simulink model "pi_seqOfFixedSizeIface"  (R2018b)
settings: Solver=FixedStepDiscrete  StartTime=0.0  StopTime=10.0  RelTol=1e-3
settings Model: Creator=matlab  LastModifiedBy=matlab
settings DataIOCC: SaveOutput=off  SignalLogging=off  SaveTime=off
settings OptimizationCC: DefaultParameterBehavior=Inlined  EnhancedBackFolding=on  PassReuseOutputArgsAs=Individual arguments  OptimizeBlockOrder=speed  DifferentSizesBufferReuse=on  OptimizationCustomize=off
settings DebuggingCC: ParameterTunabilityLossMsg=error
settings SFSimCC: MATLABDynamicMemAlloc=off
settings RTWCC: SystemTargetFile=ert.tlc  TemplateMakefile=ert_default_tmf  PostCodeGenCommand=packNGo(buildInfo);  GenerateReport=on  IncludeHyperlinkInReport=on  LaunchReport=on  GenerateTraceInfo=on  GenerateTraceReport=on  GenerateTraceReportSl=on  GenerateTraceReportSf=on  GenerateTraceReportEml=on
settings CodeAppCC: ForceParamTrailComments=on  IgnoreCustomStorageClasses=off  OperatorAnnotations=on  SimulinkDataObjDesc=on  SFDataObjDesc=on  InsertBlockDesc=on
settings ERTTargetCC: TargetLangStandard=C99 (ISO)  GenerateSampleERTMain=on  InlinedParameterPlacement=NonHierarchical  ERTCustomFileTemplate=example_file_process.tlc

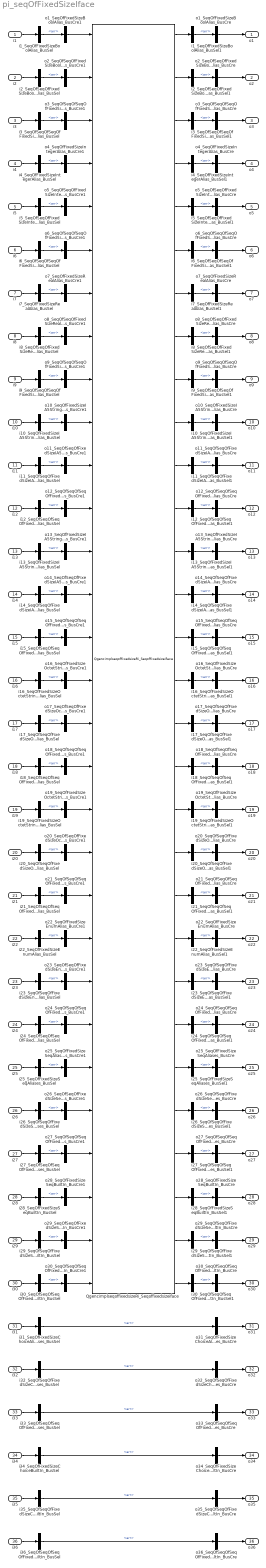
== system pi_seqOfFixedSizeIface ==
  i1 : Inport  OutDataTypeStr=Bus: SeqOfFixedSizeBoolAlias  BusOutputAsStruct=on
  i2 : Inport  Port=2  OutDataTypeStr=Bus: SeqOfSeqOfFixedSizeBoolAlias  BusOutputAsStruct=on
  i3 : Inport  Port=3  OutDataTypeStr=Bus: SeqOfSeqOfSeqOfFixedSizeBoolAlias  BusOutputAsStruct=on
  i4 : Inport  Port=4  OutDataTypeStr=Bus: SeqOfFixedSizeIntegerAlias  BusOutputAsStruct=on
  i5 : Inport  Port=5  OutDataTypeStr=Bus: SeqOfSeqOfFixedSizeIntegerAlias  BusOutputAsStruct=on
  i6 : Inport  Port=6  OutDataTypeStr=Bus: SeqOfSeqOfSeqOfFixedSizeIntegerAlias  BusOutputAsStruct=on
  i7 : Inport  Port=7  OutDataTypeStr=Bus: SeqOfFixedSizeRealAlias  BusOutputAsStruct=on
  i8 : Inport  Port=8  OutDataTypeStr=Bus: SeqOfSeqOfFixedSizeRealAlias  BusOutputAsStruct=on
  i9 : Inport  Port=9  OutDataTypeStr=Bus: SeqOfSeqOfSeqOfFixedSizeRealAlias  BusOutputAsStruct=on
  i10 : Inport  Port=10  OutDataTypeStr=Bus: SeqOfFixedSizeIA5StringFixedSizeAlias  BusOutputAsStruct=on
  i11 : Inport  Port=11  OutDataTypeStr=Bus: SeqOfSeqOfFixedSizeIA5StringFixedSizeAlias  BusOutputAsStruct=on
  i12 : Inport  Port=12  OutDataTypeStr=Bus: SeqOfSeqOfSeqOfFixedSizeIA5StringFixedSizeAlias  BusOutputAsStruct=on
  i13 : Inport  Port=13  OutDataTypeStr=Bus: SeqOfFixedSizeIA5StringVarSizeAlias  BusOutputAsStruct=on
  i14 : Inport  Port=14  OutDataTypeStr=Bus: SeqOfSeqOfFixedSizeIA5StringVarSizeAlias  BusOutputAsStruct=on
  i15 : Inport  Port=15  OutDataTypeStr=Bus: SeqOfSeqOfSeqOfFixedSizeIA5StringVarSizeAlias  BusOutputAsStruct=on
  i16 : Inport  Port=16  OutDataTypeStr=Bus: SeqOfFixedSizeOctetStringFixedSizeAlias  BusOutputAsStruct=on
  i17 : Inport  Port=17  OutDataTypeStr=Bus: SeqOfSeqOfFixedSizeOctetStringFixedSizeAlias  BusOutputAsStruct=on
  i18 : Inport  Port=18  OutDataTypeStr=Bus: SeqOfSeqOfSeqOfFixedSizeOctetStringFixedSizeAlias  BusOutputAsStruct=on
  i19 : Inport  Port=19  OutDataTypeStr=Bus: SeqOfFixedSizeOctetStringVarSizeAlias  BusOutputAsStruct=on
  i20 : Inport  Port=20  OutDataTypeStr=Bus: SeqOfSeqOfFixedSizeOctetStringVarSizeAlias  BusOutputAsStruct=on
  i21 : Inport  Port=21  OutDataTypeStr=Bus: SeqOfSeqOfSeqOfFixedSizeOctetStringVarSizeAlias  BusOutputAsStruct=on
  i22 : Inport  Port=22  OutDataTypeStr=Bus: SeqOfFixedSizeEnumAlias  BusOutputAsStruct=on
  i23 : Inport  Port=23  OutDataTypeStr=Bus: SeqOfSeqOfFixedSizeEnumAlias  BusOutputAsStruct=on
  i24 : Inport  Port=24  OutDataTypeStr=Bus: SeqOfSeqOfSeqOfFixedSizeEnumAlias  BusOutputAsStruct=on
  i25 : Inport  Port=25  OutDataTypeStr=Bus: SeqOfFixedSizeSeqAliases  BusOutputAsStruct=on
  i26 : Inport  Port=26  OutDataTypeStr=Bus: SeqOfSeqOfFixedSizeSeqAliases  BusOutputAsStruct=on
  i27 : Inport  Port=27  OutDataTypeStr=Bus: SeqOfSeqOfSeqOfFixedSizeSeqAliases  BusOutputAsStruct=on
  i28 : Inport  Port=28  OutDataTypeStr=Bus: SeqOfFixedSizeSeqBuiltIn  BusOutputAsStruct=on
  i29 : Inport  Port=29  OutDataTypeStr=Bus: SeqOfSeqOfFixedSizeSeqBuiltIn  BusOutputAsStruct=on
  i30 : Inport  Port=30  OutDataTypeStr=Bus: SeqOfSeqOfSeqOfFixedSizeSeqBuiltIn  BusOutputAsStruct=on
  i31 : Inport  Port=31  OutDataTypeStr=Bus: SeqOfFixedSizeChoiceAliases  BusOutputAsStruct=on
  i32 : Inport  Port=32  OutDataTypeStr=Bus: SeqOfSeqOfFixedSizeChoiceAliases  BusOutputAsStruct=on
  i33 : Inport  Port=33  OutDataTypeStr=Bus: SeqOfSeqOfSeqOfFixedSizeChoiceAliases  BusOutputAsStruct=on
  i34 : Inport  Port=34  OutDataTypeStr=Bus: SeqOfFixedSizeChoiceBuiltIn  BusOutputAsStruct=on
  i35 : Inport  Port=35  OutDataTypeStr=Bus: SeqOfSeqOfFixedSizeChoiceBuiltIn  BusOutputAsStruct=on
  i36 : Inport  Port=36  OutDataTypeStr=Bus: SeqOfSeqOfSeqOfFixedSizeChoiceBuiltIn  BusOutputAsStruct=on
  QgencimplseqoffixedsizeRi_Seqoffixedsizeiface : S-Function  FunctionName=QgencimplseqoffixedsizeRi_Seqoffixedsizeiface  SFunctionDeploymentMode=off  EnableBusSupport=off  mask(Legacy Function){SFunctionSpec=void qgencimplseqoffixedsize_RI_ri_seqOfFixedSizeIface(SeqOfFixedSizeBoolAlias u1[1], SeqOfSeqOfFixedSizeBoolAlias u2[1], SeqOfSeqOfSeqOfFixedSizeBoolAlias u3[1], SeqOfFixedSizeIntegerAlias u4[1], SeqOfSeqOfFixedSizeIntegerAlias u5[1], SeqOfSeqOfSeqOfFixedSizeIntegerAlias u6[1], SeqOfFixedSizeRealAlias u7[1], SeqOfSeqOfFixedSizeRealAlias u8[1], SeqOfSeqOfSeqOfFixedSizeRealAlias u9[1], SeqOfFixedSizeIA5StringFixedSizeAlias u10[1], SeqOfSeqOfFixedSizeIA5StringFixedSizeAlias u11[1], SeqOfSeqOfSeqOfFixedSizeIA5StringFixedSizeAlias u12[1], SeqOfFixedSizeIA5StringVarSizeAlias u13[1], SeqOfSeqOfFixedSizeIA5StringVarSizeAlias u14[1], SeqOfSeqOfSeqOfFixedSizeIA5StringVarSizeAlias u15[1], SeqOfFixedSizeOctetStringFixedSizeAlias u16[1], SeqOfSeqOfFixedSizeOctetStringFixedSizeAlias u17[1], SeqOfSeqOfSeqOfFixedSizeOctetStringFixedSizeAlias u18[1], SeqOfFixedSizeOctetStringVarSizeAlias u19[1], SeqOfSeqOfFixedSizeOctetStringVarSizeAlias u20[1], SeqOfSeqOfSeqOfFixedSizeOctetStringVarSizeAlias u21[1], SeqOfFixedSizeEnumAlias u22[1], SeqOfSeqOfFixedSizeEnumAlias u23[1], SeqOfSeqOfSeqOfFixedSizeEnumAlias u24[1], SeqOfFixedSizeSeqAliases u25[1], SeqOfSeqOfFixedSizeSeqAliases u26[1], SeqOfSeqOfSeqOfFixedSizeSeqAliases u27[1], SeqOfFixedSizeSeqBuiltIn u28[1], SeqOfSeqOfFixedSizeSeqBuiltIn u29[1], SeqOfSeqOfSeqOfFixedSizeSeqBuiltIn u30[1], SeqOfFixedSizeBoolAlias y1[1], SeqOfSeqOfFixedSizeBoolAlias y2[1], SeqOfSeqOfSeqOfFixedSizeBoolAlias y3[1], SeqOfFixedSizeIntegerAlias y4[1], SeqOfSeqOfFixedSizeIntegerAlias y5[1], SeqOfSeqOfSeqOfFixedSizeIntegerAlias y6[1], SeqOfFixedSizeRealAlias y7[1], SeqOfSeqOfFixedSizeRealAlias y8[1], SeqOfSeqOfSeqOfFixedSizeRealAlias y9[1], SeqOfFixedSizeIA5StringFixedSizeAlias y10[1], SeqOfSeqOfFixedSizeIA5StringFixedSizeAlias y11[1], SeqOfSeqOfSeqOfFixedSizeIA5StringFixedSizeAlias y12[1], SeqOfFixedSizeIA5StringVarSizeAlias y13[1], SeqOfSeqOfFixedSizeIA5StringVarSizeAlias y14[1], SeqOfSeqOfSeqOfFixedSizeIA5StringVarSizeAlias y15[1], SeqOfFixedSizeOctetStringFixedSizeAlias y16[1], SeqOfSeqOfFixedSizeOctetStringFixedSizeAlias y17[1], SeqOfSeqOfSeqOfFixedSizeOctetStringFixedSizeAlias y18[1], SeqOfFixedSizeOctetStringVarSizeAlias y19[1], SeqOfSeqOfFixedSizeOctetStringVarSizeAlias y20[1], SeqOfSeqOfSeqOfFixedSizeOctetStringVarSizeAlias y21[1], SeqOfFixedSizeEnumAlias y22[1], SeqOfSeqOfFixedSizeEnumAlias y23[1], SeqOfSeqOfSeqOfFixedSizeEnumAlias y24[1], SeqOfFixedSizeSeqAliases y25[1], SeqOfSeqOfFixedSizeSeqAliases y26[1], SeqOfSeqOfSeqOfFixedSizeSeqAliases y27[1], SeqOfFixedSizeSeqBuiltIn y28[1], SeqOfSeqOfFixedSizeSeqBuiltIn y29[1], SeqOfSeqOfSeqOfFixedSizeSeqBuiltIn y30[1]), ShowSpec=off}
      mask prompts: ShowSpec "Display function specification"
      mask help:
      | This block allows you to call the legacy functions specified by the following Legacy Code Tool definition:
      | def.SFunctionName = 'QgencimplseqoffixedsizeRi_Seqoffixedsizeiface';
      | def.OutputFcnSpec = 'void qgencimplseqoffixedsize_RI_ri_seqOfFixedSizeIface(SeqOfFixedSizeBoolAlias u1[1], SeqOfSeqOfFixedSizeBoolAlias u2[1], SeqOfSeqOfSeqOfFixedSizeBoolAlias u3[1], SeqOfFixedSizeIntegerAlias u4[1], SeqOfSeqOfFixedSizeIntegerAlias u5[1], SeqOfSeqOfSeqOfFixedSizeIntegerAlias u6[1], SeqOfFixedSizeRealAlias u7[1], SeqOfSeqOfFixedSizeRealAlias u8[1], SeqOfSeqOfSeqOfFixedSizeRealAlias u9[1], SeqOfFixedSizeIA5StringFixedSizeAlias u10[1], SeqOfSeqOfFixedSizeIA5StringFixedSizeAlias u11[1], SeqOfSeqOfSeqOfFixedSizeIA5StringFixedSizeAlias u12[1], SeqOfFixedSizeIA5StringVarSizeAlias u13[1], SeqOfSeqOfFixedSizeIA5StringVarSizeAlias u14[1], SeqOfSeqOfSeqOfFixedSizeIA5StringVarSizeAlias u15[1], SeqOfFixedSizeOctetStringFixedSizeAlias u16[1], SeqOfSeqOfFixedSizeOctetStringFixedSizeAlias u17[1], SeqOfSeqOfSeqOfFixedSizeOctetStringFixedSizeAlias u18[1], SeqOfFixedSizeOctetStringVarSizeAlias u19[1], SeqOfSeqOfFixedSizeOctetStringVarSizeAlias u20[1], SeqOfSeqOfSeqOfFixedSizeOctetStringVarSizeAlias u21[1], SeqOfFixedSizeEnumAlias u22[1], SeqOfSeqOfFixedSizeEnumAlias u23[1], SeqOfSeqOfSeqOfFixedSizeEnumAlias u24[1], SeqOfFixedSizeSeqAliases u25[1], SeqOfSeqOfFixedSizeSeqAliases u26[1], SeqOfSeqOfSeqOfFixedSizeSeqAliases u27[1], SeqOfFixedSizeSeqBuiltIn u28[1], SeqOfSeqOfFixedSizeSeqBuiltIn u29[1], SeqOfSeqOfSeqOfFixedSizeSeqBuiltIn u30[1], SeqOfFixedSizeBoolAlias y1[1], SeqOfSeqOfFixedSizeBoolAlias y2[1], SeqOfSeqOfSeqOfFixedSizeBoolAlias y3[1], SeqOfFixedSizeIntegerAlias y4[1], SeqOfSeqOfFixedSizeIntegerAlias y5[1], SeqOfSeqOfSeqOfFixedSizeIntegerAlias y6[1], SeqOfFixedSizeRealAlias y7[1], SeqOfSeqOfFixedSizeRealAlias y8[1], SeqOfSeqOfSeqOfFixedSizeRealAlias y9[1], SeqOfFixedSizeIA5StringFixedSizeAlias y10[1], SeqOfSeqOfFixedSizeIA5StringFixedSizeAlias y11[1], SeqOfSeqOfSeqOfFixedSizeIA5StringFixedSizeAlias y12[1], SeqOfFixedSizeIA5StringVarSizeAlias y13[1], SeqOfSeqOfFixedSizeIA5StringVarSizeAlias y14[1], SeqOfSeqOfSeqOfFixedSizeIA5StringVarSizeAlias y15[1], SeqOfFixedSizeOctetStringFixedSizeAlias y16[1], SeqOfSeqOfFixedSizeOctetStringFixedSizeAlias y17[1], SeqOfSeqOfSeqOfFixedSizeOctetStringFixedSizeAlias y18[1], SeqOfFixedSizeOctetStringVarSizeAlias y19[1], SeqOfSeqOfFixedSizeOctetStringVarSizeAlias y20[1], SeqOfSeqOfSeqOfFixedSizeOctetStringVarSizeAlias y21[1], SeqOfFixedSizeEnumAlias y22[1], SeqOfSeqOfFixedSizeEnumAlias y23[1], SeqOfSeqOfSeqOfFixedSizeEnumAlias y24[1], SeqOfFixedSizeSeqAliases y25[1], SeqOfSeqOfFixedSizeSeqAliases y26[1], SeqOfSeqOfSeqOfFixedSizeSeqAliases y27[1], SeqOfFixedSizeSeqBuiltIn y28[1], SeqOfSeqOfFixedSizeSeqBuiltIn y29[1], SeqOfSeqOfSeqOfFixedSizeSeqBuiltIn y30[1])';
      | def.HeaderFiles = {'qgencimplseqoffixedsize_invoke_ri.h'};
      | def.SourceFiles = {'qgencimplseqoffixedsize_invoke_ri.c'};
      | def.IncPaths = {'..\..\..\dataview\C'};
      mask Help: <p>This block was generated automatically by the Legacy Code Tool. For detailed help on this tool, call<a href="matlab:legacy_code('help')"> legacy_code('help')</a>.</p>
      mask Callback ShowSpec:
      | if strcmp(get_param(gcbh, 'ShowSpec'), 'on')
      |   set_param(gcbh, 'MaskDisplay', sprintf('fprintf(''%s'');', get_param(gcbh, 'SFunctionSpec')));
      | else
      |   set_param(gcbh, 'MaskDisplay', sprintf('fprintf(''%s'');', get_param(gcbh, 'FunctionName')));
      | end
      mask Display: fprintf('QgencimplseqoffixedsizeRi_Seqoffixedsizeiface');
  i10_SeqOfFixedSizeIA5StringFixedSizeAlias_BusSel : BusSelector  OutputSignals=arr
  i10_SeqOfFixedSizeIA5StringFixedSizeAlias_BusSel1 : BusSelector  OutputSignals=arr
  i11_SeqOfSeqOfFixedSizeIA5StringFixedSizeAlias_BusSel : BusSelector  OutputSignals=arr
  i11_SeqOfSeqOfFixedSizeIA5StringFixedSizeAlias_BusSel1 : BusSelector  OutputSignals=arr
  i12_SeqOfSeqOfSeqOfFixedSizeIA5StringFixedSizeAlias_BusSel : BusSelector  OutputSignals=arr
  i12_SeqOfSeqOfSeqOfFixedSizeIA5StringFixedSizeAlias_BusSel1 : BusSelector  OutputSignals=arr
  i13_SeqOfFixedSizeIA5StringVarSizeAlias_BusSel : BusSelector  OutputSignals=arr
  i13_SeqOfFixedSizeIA5StringVarSizeAlias_BusSel1 : BusSelector  OutputSignals=arr
  i14_SeqOfSeqOfFixedSizeIA5StringVarSizeAlias_BusSel : BusSelector  OutputSignals=arr
  i14_SeqOfSeqOfFixedSizeIA5StringVarSizeAlias_BusSel1 : BusSelector  OutputSignals=arr
  i15_SeqOfSeqOfSeqOfFixedSizeIA5StringVarSizeAlias_BusSel : BusSelector  OutputSignals=arr
  i15_SeqOfSeqOfSeqOfFixedSizeIA5StringVarSizeAlias_BusSel1 : BusSelector  OutputSignals=arr
  i16_SeqOfFixedSizeOctetStringFixedSizeAlias_BusSel : BusSelector  OutputSignals=arr
  i16_SeqOfFixedSizeOctetStringFixedSizeAlias_BusSel1 : BusSelector  OutputSignals=arr
  i17_SeqOfSeqOfFixedSizeOctetStringFixedSizeAlias_BusSel : BusSelector  OutputSignals=arr
  i17_SeqOfSeqOfFixedSizeOctetStringFixedSizeAlias_BusSel1 : BusSelector  OutputSignals=arr
  i18_SeqOfSeqOfSeqOfFixedSizeOctetStringFixedSizeAlias_BusSel : BusSelector  OutputSignals=arr
  i18_SeqOfSeqOfSeqOfFixedSizeOctetStringFixedSizeAlias_BusSel1 : BusSelector  OutputSignals=arr
  i19_SeqOfFixedSizeOctetStringVarSizeAlias_BusSel : BusSelector  OutputSignals=arr
  i19_SeqOfFixedSizeOctetStringVarSizeAlias_BusSel1 : BusSelector  OutputSignals=arr
  i1_SeqOfFixedSizeBoolAlias_BusSel : BusSelector  OutputSignals=arr
  i1_SeqOfFixedSizeBoolAlias_BusSel1 : BusSelector  OutputSignals=arr
  i20_SeqOfSeqOfFixedSizeOctetStringVarSizeAlias_BusSel : BusSelector  OutputSignals=arr
  i20_SeqOfSeqOfFixedSizeOctetStringVarSizeAlias_BusSel1 : BusSelector  OutputSignals=arr
  i21_SeqOfSeqOfSeqOfFixedSizeOctetStringVarSizeAlias_BusSel : BusSelector  OutputSignals=arr
  i21_SeqOfSeqOfSeqOfFixedSizeOctetStringVarSizeAlias_BusSel1 : BusSelector  OutputSignals=arr
  i22_SeqOfFixedSizeEnumAlias_BusSel : BusSelector  OutputSignals=arr
  i22_SeqOfFixedSizeEnumAlias_BusSel1 : BusSelector  OutputSignals=arr
  i23_SeqOfSeqOfFixedSizeEnumAlias_BusSel : BusSelector  OutputSignals=arr
  i23_SeqOfSeqOfFixedSizeEnumAlias_BusSel1 : BusSelector  OutputSignals=arr
  i24_SeqOfSeqOfSeqOfFixedSizeEnumAlias_BusSel : BusSelector  OutputSignals=arr
  i24_SeqOfSeqOfSeqOfFixedSizeEnumAlias_BusSel1 : BusSelector  OutputSignals=arr
  i25_SeqOfFixedSizeSeqAliases_BusSel : BusSelector  OutputSignals=arr
  i25_SeqOfFixedSizeSeqAliases_BusSel1 : BusSelector  OutputSignals=arr
  i26_SeqOfSeqOfFixedSizeSeqAliases_BusSel : BusSelector  OutputSignals=arr
  i26_SeqOfSeqOfFixedSizeSeqAliases_BusSel1 : BusSelector  OutputSignals=arr
  i27_SeqOfSeqOfSeqOfFixedSizeSeqAliases_BusSel : BusSelector  OutputSignals=arr
  i27_SeqOfSeqOfSeqOfFixedSizeSeqAliases_BusSel1 : BusSelector  OutputSignals=arr
  i28_SeqOfFixedSizeSeqBuiltIn_BusSel : BusSelector  OutputSignals=arr
  i28_SeqOfFixedSizeSeqBuiltIn_BusSel1 : BusSelector  OutputSignals=arr
  i29_SeqOfSeqOfFixedSizeSeqBuiltIn_BusSel : BusSelector  OutputSignals=arr
  i29_SeqOfSeqOfFixedSizeSeqBuiltIn_BusSel1 : BusSelector  OutputSignals=arr
  i2_SeqOfSeqOfFixedSizeBoolAlias_BusSel : BusSelector  OutputSignals=arr
  i2_SeqOfSeqOfFixedSizeBoolAlias_BusSel1 : BusSelector  OutputSignals=arr
  i30_SeqOfSeqOfSeqOfFixedSizeSeqBuiltIn_BusSel : BusSelector  OutputSignals=arr
  i30_SeqOfSeqOfSeqOfFixedSizeSeqBuiltIn_BusSel1 : BusSelector  OutputSignals=arr
  i31_SeqOfFixedSizeChoiceAliases_BusSel : BusSelector  OutputSignals=arr
  i32_SeqOfSeqOfFixedSizeChoiceAliases_BusSel : BusSelector  OutputSignals=arr
  i33_SeqOfSeqOfSeqOfFixedSizeChoiceAliases_BusSel : BusSelector  OutputSignals=arr
  i34_SeqOfFixedSizeChoiceBuiltIn_BusSel : BusSelector  OutputSignals=arr
  i35_SeqOfSeqOfFixedSizeChoiceBuiltIn_BusSel : BusSelector  OutputSignals=arr
  i36_SeqOfSeqOfSeqOfFixedSizeChoiceBuiltIn_BusSel : BusSelector  OutputSignals=arr
  i3_SeqOfSeqOfSeqOfFixedSizeBoolAlias_BusSel : BusSelector  OutputSignals=arr
  i3_SeqOfSeqOfSeqOfFixedSizeBoolAlias_BusSel1 : BusSelector  OutputSignals=arr
  i4_SeqOfFixedSizeIntegerAlias_BusSel : BusSelector  OutputSignals=arr
  i4_SeqOfFixedSizeIntegerAlias_BusSel1 : BusSelector  OutputSignals=arr
  i5_SeqOfSeqOfFixedSizeIntegerAlias_BusSel : BusSelector  OutputSignals=arr
  i5_SeqOfSeqOfFixedSizeIntegerAlias_BusSel1 : BusSelector  OutputSignals=arr
  i6_SeqOfSeqOfSeqOfFixedSizeIntegerAlias_BusSel : BusSelector  OutputSignals=arr
  i6_SeqOfSeqOfSeqOfFixedSizeIntegerAlias_BusSel1 : BusSelector  OutputSignals=arr
  i7_SeqOfFixedSizeRealAlias_BusSel : BusSelector  OutputSignals=arr
  i7_SeqOfFixedSizeRealAlias_BusSel1 : BusSelector  OutputSignals=arr
  i8_SeqOfSeqOfFixedSizeRealAlias_BusSel : BusSelector  OutputSignals=arr
  i8_SeqOfSeqOfFixedSizeRealAlias_BusSel1 : BusSelector  OutputSignals=arr
  i9_SeqOfSeqOfSeqOfFixedSizeRealAlias_BusSel : BusSelector  OutputSignals=arr
  i9_SeqOfSeqOfSeqOfFixedSizeRealAlias_BusSel1 : BusSelector  OutputSignals=arr
  o10_SeqOfFixedSizeIA5StringFixedSizeAlias_BusCre : BusCreator  Inputs=1  OutDataTypeStr=Bus: SeqOfFixedSizeIA5StringFixedSizeAlias  NonVirtualBus=on
  o10_SeqOfFixedSizeIA5StringFixedSizeAlias_BusCre1 : BusCreator  Inputs=1  OutDataTypeStr=Bus: SeqOfFixedSizeIA5StringFixedSizeAlias  NonVirtualBus=on
  o11_SeqOfSeqOfFixedSizeIA5StringFixedSizeAlias_BusCre : BusCreator  Inputs=1  OutDataTypeStr=Bus: SeqOfSeqOfFixedSizeIA5StringFixedSizeAlias  NonVirtualBus=on
  o11_SeqOfSeqOfFixedSizeIA5StringFixedSizeAlias_BusCre1 : BusCreator  Inputs=1  OutDataTypeStr=Bus: SeqOfSeqOfFixedSizeIA5StringFixedSizeAlias  NonVirtualBus=on
  o12_SeqOfSeqOfSeqOfFixedSizeIA5StringFixedSizeAlias_BusCre : BusCreator  Inputs=1  OutDataTypeStr=Bus: SeqOfSeqOfSeqOfFixedSizeIA5StringFixedSizeAlias  NonVirtualBus=on
  o12_SeqOfSeqOfSeqOfFixedSizeIA5StringFixedSizeAlias_BusCre1 : BusCreator  Inputs=1  OutDataTypeStr=Bus: SeqOfSeqOfSeqOfFixedSizeIA5StringFixedSizeAlias  NonVirtualBus=on
  o13_SeqOfFixedSizeIA5StringVarSizeAlias_BusCre : BusCreator  Inputs=1  OutDataTypeStr=Bus: SeqOfFixedSizeIA5StringVarSizeAlias  NonVirtualBus=on
  o13_SeqOfFixedSizeIA5StringVarSizeAlias_BusCre1 : BusCreator  Inputs=1  OutDataTypeStr=Bus: SeqOfFixedSizeIA5StringVarSizeAlias  NonVirtualBus=on
  o14_SeqOfSeqOfFixedSizeIA5StringVarSizeAlias_BusCre : BusCreator  Inputs=1  OutDataTypeStr=Bus: SeqOfSeqOfFixedSizeIA5StringVarSizeAlias  NonVirtualBus=on
  o14_SeqOfSeqOfFixedSizeIA5StringVarSizeAlias_BusCre1 : BusCreator  Inputs=1  OutDataTypeStr=Bus: SeqOfSeqOfFixedSizeIA5StringVarSizeAlias  NonVirtualBus=on
  o15_SeqOfSeqOfSeqOfFixedSizeIA5StringVarSizeAlias_BusCre : BusCreator  Inputs=1  OutDataTypeStr=Bus: SeqOfSeqOfSeqOfFixedSizeIA5StringVarSizeAlias  NonVirtualBus=on
  o15_SeqOfSeqOfSeqOfFixedSizeIA5StringVarSizeAlias_BusCre1 : BusCreator  Inputs=1  OutDataTypeStr=Bus: SeqOfSeqOfSeqOfFixedSizeIA5StringVarSizeAlias  NonVirtualBus=on
  o16_SeqOfFixedSizeOctetStringFixedSizeAlias_BusCre : BusCreator  Inputs=1  OutDataTypeStr=Bus: SeqOfFixedSizeOctetStringFixedSizeAlias  NonVirtualBus=on
  o16_SeqOfFixedSizeOctetStringFixedSizeAlias_BusCre1 : BusCreator  Inputs=1  OutDataTypeStr=Bus: SeqOfFixedSizeOctetStringFixedSizeAlias  NonVirtualBus=on
  o17_SeqOfSeqOfFixedSizeOctetStringFixedSizeAlias_BusCre : BusCreator  Inputs=1  OutDataTypeStr=Bus: SeqOfSeqOfFixedSizeOctetStringFixedSizeAlias  NonVirtualBus=on
  o17_SeqOfSeqOfFixedSizeOctetStringFixedSizeAlias_BusCre1 : BusCreator  Inputs=1  OutDataTypeStr=Bus: SeqOfSeqOfFixedSizeOctetStringFixedSizeAlias  NonVirtualBus=on
  o18_SeqOfSeqOfSeqOfFixedSizeOctetStringFixedSizeAlias_BusCre : BusCreator  Inputs=1  OutDataTypeStr=Bus: SeqOfSeqOfSeqOfFixedSizeOctetStringFixedSizeAlias  NonVirtualBus=on
  o18_SeqOfSeqOfSeqOfFixedSizeOctetStringFixedSizeAlias_BusCre1 : BusCreator  Inputs=1  OutDataTypeStr=Bus: SeqOfSeqOfSeqOfFixedSizeOctetStringFixedSizeAlias  NonVirtualBus=on
  o19_SeqOfFixedSizeOctetStringVarSizeAlias_BusCre : BusCreator  Inputs=1  OutDataTypeStr=Bus: SeqOfFixedSizeOctetStringVarSizeAlias  NonVirtualBus=on
  o19_SeqOfFixedSizeOctetStringVarSizeAlias_BusCre1 : BusCreator  Inputs=1  OutDataTypeStr=Bus: SeqOfFixedSizeOctetStringVarSizeAlias  NonVirtualBus=on
  o1_SeqOfFixedSizeBoolAlias_BusCre : BusCreator  Inputs=1  OutDataTypeStr=Bus: SeqOfFixedSizeBoolAlias  NonVirtualBus=on
  o1_SeqOfFixedSizeBoolAlias_BusCre1 : BusCreator  Inputs=1  OutDataTypeStr=Bus: SeqOfFixedSizeBoolAlias  NonVirtualBus=on
  o20_SeqOfSeqOfFixedSizeOctetStringVarSizeAlias_BusCre : BusCreator  Inputs=1  OutDataTypeStr=Bus: SeqOfSeqOfFixedSizeOctetStringVarSizeAlias  NonVirtualBus=on
  o20_SeqOfSeqOfFixedSizeOctetStringVarSizeAlias_BusCre1 : BusCreator  Inputs=1  OutDataTypeStr=Bus: SeqOfSeqOfFixedSizeOctetStringVarSizeAlias  NonVirtualBus=on
  o21_SeqOfSeqOfSeqOfFixedSizeOctetStringVarSizeAlias_BusCre : BusCreator  Inputs=1  OutDataTypeStr=Bus: SeqOfSeqOfSeqOfFixedSizeOctetStringVarSizeAlias  NonVirtualBus=on
  o21_SeqOfSeqOfSeqOfFixedSizeOctetStringVarSizeAlias_BusCre1 : BusCreator  Inputs=1  OutDataTypeStr=Bus: SeqOfSeqOfSeqOfFixedSizeOctetStringVarSizeAlias  NonVirtualBus=on
  o22_SeqOfFixedSizeEnumAlias_BusCre : BusCreator  Inputs=1  OutDataTypeStr=Bus: SeqOfFixedSizeEnumAlias  NonVirtualBus=on
  o22_SeqOfFixedSizeEnumAlias_BusCre1 : BusCreator  Inputs=1  OutDataTypeStr=Bus: SeqOfFixedSizeEnumAlias  NonVirtualBus=on
  o23_SeqOfSeqOfFixedSizeEnumAlias_BusCre : BusCreator  Inputs=1  OutDataTypeStr=Bus: SeqOfSeqOfFixedSizeEnumAlias  NonVirtualBus=on
  o23_SeqOfSeqOfFixedSizeEnumAlias_BusCre1 : BusCreator  Inputs=1  OutDataTypeStr=Bus: SeqOfSeqOfFixedSizeEnumAlias  NonVirtualBus=on
  o24_SeqOfSeqOfSeqOfFixedSizeEnumAlias_BusCre : BusCreator  Inputs=1  OutDataTypeStr=Bus: SeqOfSeqOfSeqOfFixedSizeEnumAlias  NonVirtualBus=on
  o24_SeqOfSeqOfSeqOfFixedSizeEnumAlias_BusCre1 : BusCreator  Inputs=1  OutDataTypeStr=Bus: SeqOfSeqOfSeqOfFixedSizeEnumAlias  NonVirtualBus=on
  o25_SeqOfFixedSizeSeqAliases_BusCre : BusCreator  Inputs=1  OutDataTypeStr=Bus: SeqOfFixedSizeSeqAliases  NonVirtualBus=on
  o25_SeqOfFixedSizeSeqAliases_BusCre1 : BusCreator  Inputs=1  OutDataTypeStr=Bus: SeqOfFixedSizeSeqAliases  NonVirtualBus=on
  o26_SeqOfSeqOfFixedSizeSeqAliases_BusCre : BusCreator  Inputs=1  OutDataTypeStr=Bus: SeqOfSeqOfFixedSizeSeqAliases  NonVirtualBus=on
  o26_SeqOfSeqOfFixedSizeSeqAliases_BusCre1 : BusCreator  Inputs=1  OutDataTypeStr=Bus: SeqOfSeqOfFixedSizeSeqAliases  NonVirtualBus=on
  o27_SeqOfSeqOfSeqOfFixedSizeSeqAliases_BusCre : BusCreator  Inputs=1  OutDataTypeStr=Bus: SeqOfSeqOfSeqOfFixedSizeSeqAliases  NonVirtualBus=on
  o27_SeqOfSeqOfSeqOfFixedSizeSeqAliases_BusCre1 : BusCreator  Inputs=1  OutDataTypeStr=Bus: SeqOfSeqOfSeqOfFixedSizeSeqAliases  NonVirtualBus=on
  o28_SeqOfFixedSizeSeqBuiltIn_BusCre : BusCreator  Inputs=1  OutDataTypeStr=Bus: SeqOfFixedSizeSeqBuiltIn  NonVirtualBus=on
  o28_SeqOfFixedSizeSeqBuiltIn_BusCre1 : BusCreator  Inputs=1  OutDataTypeStr=Bus: SeqOfFixedSizeSeqBuiltIn  NonVirtualBus=on
  o29_SeqOfSeqOfFixedSizeSeqBuiltIn_BusCre : BusCreator  Inputs=1  OutDataTypeStr=Bus: SeqOfSeqOfFixedSizeSeqBuiltIn  NonVirtualBus=on
  o29_SeqOfSeqOfFixedSizeSeqBuiltIn_BusCre1 : BusCreator  Inputs=1  OutDataTypeStr=Bus: SeqOfSeqOfFixedSizeSeqBuiltIn  NonVirtualBus=on
  o2_SeqOfSeqOfFixedSizeBoolAlias_BusCre : BusCreator  Inputs=1  OutDataTypeStr=Bus: SeqOfSeqOfFixedSizeBoolAlias  NonVirtualBus=on
  o2_SeqOfSeqOfFixedSizeBoolAlias_BusCre1 : BusCreator  Inputs=1  OutDataTypeStr=Bus: SeqOfSeqOfFixedSizeBoolAlias  NonVirtualBus=on
  o30_SeqOfSeqOfSeqOfFixedSizeSeqBuiltIn_BusCre : BusCreator  Inputs=1  OutDataTypeStr=Bus: SeqOfSeqOfSeqOfFixedSizeSeqBuiltIn  NonVirtualBus=on
  o30_SeqOfSeqOfSeqOfFixedSizeSeqBuiltIn_BusCre1 : BusCreator  Inputs=1  OutDataTypeStr=Bus: SeqOfSeqOfSeqOfFixedSizeSeqBuiltIn  NonVirtualBus=on
  o31_SeqOfFixedSizeChoiceAliases_BusCre : BusCreator  Inputs=1  OutDataTypeStr=Bus: SeqOfFixedSizeChoiceAliases  NonVirtualBus=on
  o32_SeqOfSeqOfFixedSizeChoiceAliases_BusCre : BusCreator  Inputs=1  OutDataTypeStr=Bus: SeqOfSeqOfFixedSizeChoiceAliases  NonVirtualBus=on
  o33_SeqOfSeqOfSeqOfFixedSizeChoiceAliases_BusCre : BusCreator  Inputs=1  OutDataTypeStr=Bus: SeqOfSeqOfSeqOfFixedSizeChoiceAliases  NonVirtualBus=on
  o34_SeqOfFixedSizeChoiceBuiltIn_BusCre : BusCreator  Inputs=1  OutDataTypeStr=Bus: SeqOfFixedSizeChoiceBuiltIn  NonVirtualBus=on
  o35_SeqOfSeqOfFixedSizeChoiceBuiltIn_BusCre : BusCreator  Inputs=1  OutDataTypeStr=Bus: SeqOfSeqOfFixedSizeChoiceBuiltIn  NonVirtualBus=on
  o36_SeqOfSeqOfSeqOfFixedSizeChoiceBuiltIn_BusCre : BusCreator  Inputs=1  OutDataTypeStr=Bus: SeqOfSeqOfSeqOfFixedSizeChoiceBuiltIn  NonVirtualBus=on
  o3_SeqOfSeqOfSeqOfFixedSizeBoolAlias_BusCre : BusCreator  Inputs=1  OutDataTypeStr=Bus: SeqOfSeqOfSeqOfFixedSizeBoolAlias  NonVirtualBus=on
  o3_SeqOfSeqOfSeqOfFixedSizeBoolAlias_BusCre1 : BusCreator  Inputs=1  OutDataTypeStr=Bus: SeqOfSeqOfSeqOfFixedSizeBoolAlias  NonVirtualBus=on
  o4_SeqOfFixedSizeIntegerAlias_BusCre : BusCreator  Inputs=1  OutDataTypeStr=Bus: SeqOfFixedSizeIntegerAlias  NonVirtualBus=on
  o4_SeqOfFixedSizeIntegerAlias_BusCre1 : BusCreator  Inputs=1  OutDataTypeStr=Bus: SeqOfFixedSizeIntegerAlias  NonVirtualBus=on
  o5_SeqOfSeqOfFixedSizeIntegerAlias_BusCre : BusCreator  Inputs=1  OutDataTypeStr=Bus: SeqOfSeqOfFixedSizeIntegerAlias  NonVirtualBus=on
  o5_SeqOfSeqOfFixedSizeIntegerAlias_BusCre1 : BusCreator  Inputs=1  OutDataTypeStr=Bus: SeqOfSeqOfFixedSizeIntegerAlias  NonVirtualBus=on
  o6_SeqOfSeqOfSeqOfFixedSizeIntegerAlias_BusCre : BusCreator  Inputs=1  OutDataTypeStr=Bus: SeqOfSeqOfSeqOfFixedSizeIntegerAlias  NonVirtualBus=on
  o6_SeqOfSeqOfSeqOfFixedSizeIntegerAlias_BusCre1 : BusCreator  Inputs=1  OutDataTypeStr=Bus: SeqOfSeqOfSeqOfFixedSizeIntegerAlias  NonVirtualBus=on
  o7_SeqOfFixedSizeRealAlias_BusCre : BusCreator  Inputs=1  OutDataTypeStr=Bus: SeqOfFixedSizeRealAlias  NonVirtualBus=on
  o7_SeqOfFixedSizeRealAlias_BusCre1 : BusCreator  Inputs=1  OutDataTypeStr=Bus: SeqOfFixedSizeRealAlias  NonVirtualBus=on
  o8_SeqOfSeqOfFixedSizeRealAlias_BusCre : BusCreator  Inputs=1  OutDataTypeStr=Bus: SeqOfSeqOfFixedSizeRealAlias  NonVirtualBus=on
  o8_SeqOfSeqOfFixedSizeRealAlias_BusCre1 : BusCreator  Inputs=1  OutDataTypeStr=Bus: SeqOfSeqOfFixedSizeRealAlias  NonVirtualBus=on
  o9_SeqOfSeqOfSeqOfFixedSizeRealAlias_BusCre : BusCreator  Inputs=1  OutDataTypeStr=Bus: SeqOfSeqOfSeqOfFixedSizeRealAlias  NonVirtualBus=on
  o9_SeqOfSeqOfSeqOfFixedSizeRealAlias_BusCre1 : BusCreator  Inputs=1  OutDataTypeStr=Bus: SeqOfSeqOfSeqOfFixedSizeRealAlias  NonVirtualBus=on
  o1 : Outport  OutDataTypeStr=Bus: SeqOfFixedSizeBoolAlias  BusOutputAsStruct=on
  o2 : Outport  Port=2  OutDataTypeStr=Bus: SeqOfSeqOfFixedSizeBoolAlias  BusOutputAsStruct=on
  o3 : Outport  Port=3  OutDataTypeStr=Bus: SeqOfSeqOfSeqOfFixedSizeBoolAlias  BusOutputAsStruct=on
  o4 : Outport  Port=4  OutDataTypeStr=Bus: SeqOfFixedSizeIntegerAlias  BusOutputAsStruct=on
  o5 : Outport  Port=5  OutDataTypeStr=Bus: SeqOfSeqOfFixedSizeIntegerAlias  BusOutputAsStruct=on
  o6 : Outport  Port=6  OutDataTypeStr=Bus: SeqOfSeqOfSeqOfFixedSizeIntegerAlias  BusOutputAsStruct=on
  o7 : Outport  Port=7  OutDataTypeStr=Bus: SeqOfFixedSizeRealAlias  BusOutputAsStruct=on
  o8 : Outport  Port=8  OutDataTypeStr=Bus: SeqOfSeqOfFixedSizeRealAlias  BusOutputAsStruct=on
  o9 : Outport  Port=9  OutDataTypeStr=Bus: SeqOfSeqOfSeqOfFixedSizeRealAlias  BusOutputAsStruct=on
  o10 : Outport  Port=10  OutDataTypeStr=Bus: SeqOfFixedSizeIA5StringFixedSizeAlias  BusOutputAsStruct=on
  o11 : Outport  Port=11  OutDataTypeStr=Bus: SeqOfSeqOfFixedSizeIA5StringFixedSizeAlias  BusOutputAsStruct=on
  o12 : Outport  Port=12  OutDataTypeStr=Bus: SeqOfSeqOfSeqOfFixedSizeIA5StringFixedSizeAlias  BusOutputAsStruct=on
  o13 : Outport  Port=13  OutDataTypeStr=Bus: SeqOfFixedSizeIA5StringVarSizeAlias  BusOutputAsStruct=on
  o14 : Outport  Port=14  OutDataTypeStr=Bus: SeqOfSeqOfFixedSizeIA5StringVarSizeAlias  BusOutputAsStruct=on
  o15 : Outport  Port=15  OutDataTypeStr=Bus: SeqOfSeqOfSeqOfFixedSizeIA5StringVarSizeAlias  BusOutputAsStruct=on
  o16 : Outport  Port=16  OutDataTypeStr=Bus: SeqOfFixedSizeOctetStringFixedSizeAlias  BusOutputAsStruct=on
  o17 : Outport  Port=17  OutDataTypeStr=Bus: SeqOfSeqOfFixedSizeOctetStringFixedSizeAlias  BusOutputAsStruct=on
  o18 : Outport  Port=18  OutDataTypeStr=Bus: SeqOfSeqOfSeqOfFixedSizeOctetStringFixedSizeAlias  BusOutputAsStruct=on
  o19 : Outport  Port=19  OutDataTypeStr=Bus: SeqOfFixedSizeOctetStringVarSizeAlias  BusOutputAsStruct=on
  o20 : Outport  Port=20  OutDataTypeStr=Bus: SeqOfSeqOfFixedSizeOctetStringVarSizeAlias  BusOutputAsStruct=on
  o21 : Outport  Port=21  OutDataTypeStr=Bus: SeqOfSeqOfSeqOfFixedSizeOctetStringVarSizeAlias  BusOutputAsStruct=on
  o22 : Outport  Port=22  OutDataTypeStr=Bus: SeqOfFixedSizeEnumAlias  BusOutputAsStruct=on
  o23 : Outport  Port=23  OutDataTypeStr=Bus: SeqOfSeqOfFixedSizeEnumAlias  BusOutputAsStruct=on
  o24 : Outport  Port=24  OutDataTypeStr=Bus: SeqOfSeqOfSeqOfFixedSizeEnumAlias  BusOutputAsStruct=on
  o25 : Outport  Port=25  OutDataTypeStr=Bus: SeqOfFixedSizeSeqAliases  BusOutputAsStruct=on
  o26 : Outport  Port=26  OutDataTypeStr=Bus: SeqOfSeqOfFixedSizeSeqAliases  BusOutputAsStruct=on
  o27 : Outport  Port=27  OutDataTypeStr=Bus: SeqOfSeqOfSeqOfFixedSizeSeqAliases  BusOutputAsStruct=on
  o28 : Outport  Port=28  OutDataTypeStr=Bus: SeqOfFixedSizeSeqBuiltIn  BusOutputAsStruct=on
  o29 : Outport  Port=29  OutDataTypeStr=Bus: SeqOfSeqOfFixedSizeSeqBuiltIn  BusOutputAsStruct=on
  o30 : Outport  Port=30  OutDataTypeStr=Bus: SeqOfSeqOfSeqOfFixedSizeSeqBuiltIn  BusOutputAsStruct=on
  o31 : Outport  Port=31  OutDataTypeStr=Bus: SeqOfFixedSizeChoiceAliases  BusOutputAsStruct=on
  o32 : Outport  Port=32  OutDataTypeStr=Bus: SeqOfSeqOfFixedSizeChoiceAliases  BusOutputAsStruct=on
  o33 : Outport  Port=33  OutDataTypeStr=Bus: SeqOfSeqOfSeqOfFixedSizeChoiceAliases  BusOutputAsStruct=on
  o34 : Outport  Port=34  OutDataTypeStr=Bus: SeqOfFixedSizeChoiceBuiltIn  BusOutputAsStruct=on
  o35 : Outport  Port=35  OutDataTypeStr=Bus: SeqOfSeqOfFixedSizeChoiceBuiltIn  BusOutputAsStruct=on
  o36 : Outport  Port=36  OutDataTypeStr=Bus: SeqOfSeqOfSeqOfFixedSizeChoiceBuiltIn  BusOutputAsStruct=on
  wires:
  i1/1 -> i1_SeqOfFixedSizeBoolAlias_BusSel/1
  i2/1 -> i2_SeqOfSeqOfFixedSizeBoolAlias_BusSel/1
  i3/1 -> i3_SeqOfSeqOfSeqOfFixedSizeBoolAlias_BusSel/1
  i4/1 -> i4_SeqOfFixedSizeIntegerAlias_BusSel/1
  i5/1 -> i5_SeqOfSeqOfFixedSizeIntegerAlias_BusSel/1
  i6/1 -> i6_SeqOfSeqOfSeqOfFixedSizeIntegerAlias_BusSel/1
  i7/1 -> i7_SeqOfFixedSizeRealAlias_BusSel/1
  i8/1 -> i8_SeqOfSeqOfFixedSizeRealAlias_BusSel/1
  i9/1 -> i9_SeqOfSeqOfSeqOfFixedSizeRealAlias_BusSel/1
  i10/1 -> i10_SeqOfFixedSizeIA5StringFixedSizeAlias_BusSel/1
  i11/1 -> i11_SeqOfSeqOfFixedSizeIA5StringFixedSizeAlias_BusSel/1
  i12/1 -> i12_SeqOfSeqOfSeqOfFixedSizeIA5StringFixedSizeAlias_BusSel/1
  i13/1 -> i13_SeqOfFixedSizeIA5StringVarSizeAlias_BusSel/1
  i14/1 -> i14_SeqOfSeqOfFixedSizeIA5StringVarSizeAlias_BusSel/1
  i15/1 -> i15_SeqOfSeqOfSeqOfFixedSizeIA5StringVarSizeAlias_BusSel/1
  i16/1 -> i16_SeqOfFixedSizeOctetStringFixedSizeAlias_BusSel/1
  i17/1 -> i17_SeqOfSeqOfFixedSizeOctetStringFixedSizeAlias_BusSel/1
  i18/1 -> i18_SeqOfSeqOfSeqOfFixedSizeOctetStringFixedSizeAlias_BusSel/1
  i19/1 -> i19_SeqOfFixedSizeOctetStringVarSizeAlias_BusSel/1
  i20/1 -> i20_SeqOfSeqOfFixedSizeOctetStringVarSizeAlias_BusSel/1
  i21/1 -> i21_SeqOfSeqOfSeqOfFixedSizeOctetStringVarSizeAlias_BusSel/1
  i22/1 -> i22_SeqOfFixedSizeEnumAlias_BusSel/1
  i23/1 -> i23_SeqOfSeqOfFixedSizeEnumAlias_BusSel/1
  i24/1 -> i24_SeqOfSeqOfSeqOfFixedSizeEnumAlias_BusSel/1
  i25/1 -> i25_SeqOfFixedSizeSeqAliases_BusSel/1
  i26/1 -> i26_SeqOfSeqOfFixedSizeSeqAliases_BusSel/1
  i27/1 -> i27_SeqOfSeqOfSeqOfFixedSizeSeqAliases_BusSel/1
  i28/1 -> i28_SeqOfFixedSizeSeqBuiltIn_BusSel/1
  i29/1 -> i29_SeqOfSeqOfFixedSizeSeqBuiltIn_BusSel/1
  i30/1 -> i30_SeqOfSeqOfSeqOfFixedSizeSeqBuiltIn_BusSel/1
  i31/1 -> i31_SeqOfFixedSizeChoiceAliases_BusSel/1
  i32/1 -> i32_SeqOfSeqOfFixedSizeChoiceAliases_BusSel/1
  i33/1 -> i33_SeqOfSeqOfSeqOfFixedSizeChoiceAliases_BusSel/1
  i34/1 -> i34_SeqOfFixedSizeChoiceBuiltIn_BusSel/1
  i35/1 -> i35_SeqOfSeqOfFixedSizeChoiceBuiltIn_BusSel/1
  i36/1 -> i36_SeqOfSeqOfSeqOfFixedSizeChoiceBuiltIn_BusSel/1
  o1_SeqOfFixedSizeBoolAlias_BusCre/1 -> o1/1
  o2_SeqOfSeqOfFixedSizeBoolAlias_BusCre/1 -> o2/1
  o3_SeqOfSeqOfSeqOfFixedSizeBoolAlias_BusCre/1 -> o3/1
  o4_SeqOfFixedSizeIntegerAlias_BusCre/1 -> o4/1
  o5_SeqOfSeqOfFixedSizeIntegerAlias_BusCre/1 -> o5/1
  o6_SeqOfSeqOfSeqOfFixedSizeIntegerAlias_BusCre/1 -> o6/1
  o7_SeqOfFixedSizeRealAlias_BusCre/1 -> o7/1
  o8_SeqOfSeqOfFixedSizeRealAlias_BusCre/1 -> o8/1
  o9_SeqOfSeqOfSeqOfFixedSizeRealAlias_BusCre/1 -> o9/1
  o10_SeqOfFixedSizeIA5StringFixedSizeAlias_BusCre/1 -> o10/1
  o11_SeqOfSeqOfFixedSizeIA5StringFixedSizeAlias_BusCre/1 -> o11/1
  o12_SeqOfSeqOfSeqOfFixedSizeIA5StringFixedSizeAlias_BusCre/1 -> o12/1
  o13_SeqOfFixedSizeIA5StringVarSizeAlias_BusCre/1 -> o13/1
  o14_SeqOfSeqOfFixedSizeIA5StringVarSizeAlias_BusCre/1 -> o14/1
  o15_SeqOfSeqOfSeqOfFixedSizeIA5StringVarSizeAlias_BusCre/1 -> o15/1
  o16_SeqOfFixedSizeOctetStringFixedSizeAlias_BusCre/1 -> o16/1
  o17_SeqOfSeqOfFixedSizeOctetStringFixedSizeAlias_BusCre/1 -> o17/1
  o18_SeqOfSeqOfSeqOfFixedSizeOctetStringFixedSizeAlias_BusCre/1 -> o18/1
  o19_SeqOfFixedSizeOctetStringVarSizeAlias_BusCre/1 -> o19/1
  o20_SeqOfSeqOfFixedSizeOctetStringVarSizeAlias_BusCre/1 -> o20/1
  o21_SeqOfSeqOfSeqOfFixedSizeOctetStringVarSizeAlias_BusCre/1 -> o21/1
  o22_SeqOfFixedSizeEnumAlias_BusCre/1 -> o22/1
  o23_SeqOfSeqOfFixedSizeEnumAlias_BusCre/1 -> o23/1
  o24_SeqOfSeqOfSeqOfFixedSizeEnumAlias_BusCre/1 -> o24/1
  o25_SeqOfFixedSizeSeqAliases_BusCre/1 -> o25/1
  o26_SeqOfSeqOfFixedSizeSeqAliases_BusCre/1 -> o26/1
  o27_SeqOfSeqOfSeqOfFixedSizeSeqAliases_BusCre/1 -> o27/1
  o28_SeqOfFixedSizeSeqBuiltIn_BusCre/1 -> o28/1
  o29_SeqOfSeqOfFixedSizeSeqBuiltIn_BusCre/1 -> o29/1
  o30_SeqOfSeqOfSeqOfFixedSizeSeqBuiltIn_BusCre/1 -> o30/1
  o31_SeqOfFixedSizeChoiceAliases_BusCre/1 -> o31/1
  o32_SeqOfSeqOfFixedSizeChoiceAliases_BusCre/1 -> o32/1
  o33_SeqOfSeqOfSeqOfFixedSizeChoiceAliases_BusCre/1 -> o33/1
  o34_SeqOfFixedSizeChoiceBuiltIn_BusCre/1 -> o34/1
  o35_SeqOfSeqOfFixedSizeChoiceBuiltIn_BusCre/1 -> o35/1
  o36_SeqOfSeqOfSeqOfFixedSizeChoiceBuiltIn_BusCre/1 -> o36/1
  o5_SeqOfSeqOfFixedSizeIntegerAlias_BusCre1/1 -> QgencimplseqoffixedsizeRi_Seqoffixedsizeiface/5
  o7_SeqOfFixedSizeRealAlias_BusCre1/1 -> QgencimplseqoffixedsizeRi_Seqoffixedsizeiface/7
  o14_SeqOfSeqOfFixedSizeIA5StringVarSizeAlias_BusCre1/1 -> QgencimplseqoffixedsizeRi_Seqoffixedsizeiface/14
  o24_SeqOfSeqOfSeqOfFixedSizeEnumAlias_BusCre1/1 -> QgencimplseqoffixedsizeRi_Seqoffixedsizeiface/24
  o3_SeqOfSeqOfSeqOfFixedSizeBoolAlias_BusCre1/1 -> QgencimplseqoffixedsizeRi_Seqoffixedsizeiface/3
  o4_SeqOfFixedSizeIntegerAlias_BusCre1/1 -> QgencimplseqoffixedsizeRi_Seqoffixedsizeiface/4
  o27_SeqOfSeqOfSeqOfFixedSizeSeqAliases_BusCre1/1 -> QgencimplseqoffixedsizeRi_Seqoffixedsizeiface/27
  o17_SeqOfSeqOfFixedSizeOctetStringFixedSizeAlias_BusCre1/1 -> QgencimplseqoffixedsizeRi_Seqoffixedsizeiface/17
  o30_SeqOfSeqOfSeqOfFixedSizeSeqBuiltIn_BusCre1/1 -> QgencimplseqoffixedsizeRi_Seqoffixedsizeiface/30
  o28_SeqOfFixedSizeSeqBuiltIn_BusCre1/1 -> QgencimplseqoffixedsizeRi_Seqoffixedsizeiface/28
  o18_SeqOfSeqOfSeqOfFixedSizeOctetStringFixedSizeAlias_BusCre1/1 -> QgencimplseqoffixedsizeRi_Seqoffixedsizeiface/18
  o29_SeqOfSeqOfFixedSizeSeqBuiltIn_BusCre1/1 -> QgencimplseqoffixedsizeRi_Seqoffixedsizeiface/29
  o26_SeqOfSeqOfFixedSizeSeqAliases_BusCre1/1 -> QgencimplseqoffixedsizeRi_Seqoffixedsizeiface/26
  o11_SeqOfSeqOfFixedSizeIA5StringFixedSizeAlias_BusCre1/1 -> QgencimplseqoffixedsizeRi_Seqoffixedsizeiface/11
  o8_SeqOfSeqOfFixedSizeRealAlias_BusCre1/1 -> QgencimplseqoffixedsizeRi_Seqoffixedsizeiface/8
  o13_SeqOfFixedSizeIA5StringVarSizeAlias_BusCre1/1 -> QgencimplseqoffixedsizeRi_Seqoffixedsizeiface/13
  o12_SeqOfSeqOfSeqOfFixedSizeIA5StringFixedSizeAlias_BusCre1/1 -> QgencimplseqoffixedsizeRi_Seqoffixedsizeiface/12
  o6_SeqOfSeqOfSeqOfFixedSizeIntegerAlias_BusCre1/1 -> QgencimplseqoffixedsizeRi_Seqoffixedsizeiface/6
  o23_SeqOfSeqOfFixedSizeEnumAlias_BusCre1/1 -> QgencimplseqoffixedsizeRi_Seqoffixedsizeiface/23
  o2_SeqOfSeqOfFixedSizeBoolAlias_BusCre1/1 -> QgencimplseqoffixedsizeRi_Seqoffixedsizeiface/2
  o10_SeqOfFixedSizeIA5StringFixedSizeAlias_BusCre1/1 -> QgencimplseqoffixedsizeRi_Seqoffixedsizeiface/10
  o1_SeqOfFixedSizeBoolAlias_BusCre1/1 -> QgencimplseqoffixedsizeRi_Seqoffixedsizeiface/1
  o19_SeqOfFixedSizeOctetStringVarSizeAlias_BusCre1/1 -> QgencimplseqoffixedsizeRi_Seqoffixedsizeiface/19
  o9_SeqOfSeqOfSeqOfFixedSizeRealAlias_BusCre1/1 -> QgencimplseqoffixedsizeRi_Seqoffixedsizeiface/9
  o22_SeqOfFixedSizeEnumAlias_BusCre1/1 -> QgencimplseqoffixedsizeRi_Seqoffixedsizeiface/22
  o16_SeqOfFixedSizeOctetStringFixedSizeAlias_BusCre1/1 -> QgencimplseqoffixedsizeRi_Seqoffixedsizeiface/16
  o20_SeqOfSeqOfFixedSizeOctetStringVarSizeAlias_BusCre1/1 -> QgencimplseqoffixedsizeRi_Seqoffixedsizeiface/20
  o15_SeqOfSeqOfSeqOfFixedSizeIA5StringVarSizeAlias_BusCre1/1 -> QgencimplseqoffixedsizeRi_Seqoffixedsizeiface/15
  o25_SeqOfFixedSizeSeqAliases_BusCre1/1 -> QgencimplseqoffixedsizeRi_Seqoffixedsizeiface/25
  o21_SeqOfSeqOfSeqOfFixedSizeOctetStringVarSizeAlias_BusCre1/1 -> QgencimplseqoffixedsizeRi_Seqoffixedsizeiface/21
  i1_SeqOfFixedSizeBoolAlias_BusSel/1 -> o1_SeqOfFixedSizeBoolAlias_BusCre1/1  "<arr>"
  i2_SeqOfSeqOfFixedSizeBoolAlias_BusSel/1 -> o2_SeqOfSeqOfFixedSizeBoolAlias_BusCre1/1  "<arr>"
  i3_SeqOfSeqOfSeqOfFixedSizeBoolAlias_BusSel/1 -> o3_SeqOfSeqOfSeqOfFixedSizeBoolAlias_BusCre1/1  "<arr>"
  i4_SeqOfFixedSizeIntegerAlias_BusSel/1 -> o4_SeqOfFixedSizeIntegerAlias_BusCre1/1  "<arr>"
  i5_SeqOfSeqOfFixedSizeIntegerAlias_BusSel/1 -> o5_SeqOfSeqOfFixedSizeIntegerAlias_BusCre1/1  "<arr>"
  i6_SeqOfSeqOfSeqOfFixedSizeIntegerAlias_BusSel/1 -> o6_SeqOfSeqOfSeqOfFixedSizeIntegerAlias_BusCre1/1  "<arr>"
  i7_SeqOfFixedSizeRealAlias_BusSel/1 -> o7_SeqOfFixedSizeRealAlias_BusCre1/1  "<arr>"
  i8_SeqOfSeqOfFixedSizeRealAlias_BusSel/1 -> o8_SeqOfSeqOfFixedSizeRealAlias_BusCre1/1  "<arr>"
  i9_SeqOfSeqOfSeqOfFixedSizeRealAlias_BusSel/1 -> o9_SeqOfSeqOfSeqOfFixedSizeRealAlias_BusCre1/1  "<arr>"
  i10_SeqOfFixedSizeIA5StringFixedSizeAlias_BusSel/1 -> o10_SeqOfFixedSizeIA5StringFixedSizeAlias_BusCre1/1  "<arr>"
  i11_SeqOfSeqOfFixedSizeIA5StringFixedSizeAlias_BusSel/1 -> o11_SeqOfSeqOfFixedSizeIA5StringFixedSizeAlias_BusCre1/1  "<arr>"
  i12_SeqOfSeqOfSeqOfFixedSizeIA5StringFixedSizeAlias_BusSel/1 -> o12_SeqOfSeqOfSeqOfFixedSizeIA5StringFixedSizeAlias_BusCre1/1  "<arr>"
  i13_SeqOfFixedSizeIA5StringVarSizeAlias_BusSel/1 -> o13_SeqOfFixedSizeIA5StringVarSizeAlias_BusCre1/1  "<arr>"
  i14_SeqOfSeqOfFixedSizeIA5StringVarSizeAlias_BusSel/1 -> o14_SeqOfSeqOfFixedSizeIA5StringVarSizeAlias_BusCre1/1  "<arr>"
  i15_SeqOfSeqOfSeqOfFixedSizeIA5StringVarSizeAlias_BusSel/1 -> o15_SeqOfSeqOfSeqOfFixedSizeIA5StringVarSizeAlias_BusCre1/1  "<arr>"
  i16_SeqOfFixedSizeOctetStringFixedSizeAlias_BusSel/1 -> o16_SeqOfFixedSizeOctetStringFixedSizeAlias_BusCre1/1  "<arr>"
  i17_SeqOfSeqOfFixedSizeOctetStringFixedSizeAlias_BusSel/1 -> o17_SeqOfSeqOfFixedSizeOctetStringFixedSizeAlias_BusCre1/1  "<arr>"
  i18_SeqOfSeqOfSeqOfFixedSizeOctetStringFixedSizeAlias_BusSel/1 -> o18_SeqOfSeqOfSeqOfFixedSizeOctetStringFixedSizeAlias_BusCre1/1  "<arr>"
  i19_SeqOfFixedSizeOctetStringVarSizeAlias_BusSel/1 -> o19_SeqOfFixedSizeOctetStringVarSizeAlias_BusCre1/1  "<arr>"
  i20_SeqOfSeqOfFixedSizeOctetStringVarSizeAlias_BusSel/1 -> o20_SeqOfSeqOfFixedSizeOctetStringVarSizeAlias_BusCre1/1  "<arr>"
  i21_SeqOfSeqOfSeqOfFixedSizeOctetStringVarSizeAlias_BusSel/1 -> o21_SeqOfSeqOfSeqOfFixedSizeOctetStringVarSizeAlias_BusCre1/1  "<arr>"
  i22_SeqOfFixedSizeEnumAlias_BusSel/1 -> o22_SeqOfFixedSizeEnumAlias_BusCre1/1  "<arr>"
  i23_SeqOfSeqOfFixedSizeEnumAlias_BusSel/1 -> o23_SeqOfSeqOfFixedSizeEnumAlias_BusCre1/1  "<arr>"
  i24_SeqOfSeqOfSeqOfFixedSizeEnumAlias_BusSel/1 -> o24_SeqOfSeqOfSeqOfFixedSizeEnumAlias_BusCre1/1  "<arr>"
  i25_SeqOfFixedSizeSeqAliases_BusSel/1 -> o25_SeqOfFixedSizeSeqAliases_BusCre1/1  "<arr>"
  i26_SeqOfSeqOfFixedSizeSeqAliases_BusSel/1 -> o26_SeqOfSeqOfFixedSizeSeqAliases_BusCre1/1  "<arr>"
  i27_SeqOfSeqOfSeqOfFixedSizeSeqAliases_BusSel/1 -> o27_SeqOfSeqOfSeqOfFixedSizeSeqAliases_BusCre1/1  "<arr>"
  i28_SeqOfFixedSizeSeqBuiltIn_BusSel/1 -> o28_SeqOfFixedSizeSeqBuiltIn_BusCre1/1  "<arr>"
  i29_SeqOfSeqOfFixedSizeSeqBuiltIn_BusSel/1 -> o29_SeqOfSeqOfFixedSizeSeqBuiltIn_BusCre1/1  "<arr>"
  i30_SeqOfSeqOfSeqOfFixedSizeSeqBuiltIn_BusSel/1 -> o30_SeqOfSeqOfSeqOfFixedSizeSeqBuiltIn_BusCre1/1  "<arr>"
  i31_SeqOfFixedSizeChoiceAliases_BusSel/1 -> o31_SeqOfFixedSizeChoiceAliases_BusCre/1  "<arr>"
  i32_SeqOfSeqOfFixedSizeChoiceAliases_BusSel/1 -> o32_SeqOfSeqOfFixedSizeChoiceAliases_BusCre/1  "<arr>"
  i34_SeqOfFixedSizeChoiceBuiltIn_BusSel/1 -> o34_SeqOfFixedSizeChoiceBuiltIn_BusCre/1  "<arr>"
  i33_SeqOfSeqOfSeqOfFixedSizeChoiceAliases_BusSel/1 -> o33_SeqOfSeqOfSeqOfFixedSizeChoiceAliases_BusCre/1  "<arr>"
  i35_SeqOfSeqOfFixedSizeChoiceBuiltIn_BusSel/1 -> o35_SeqOfSeqOfFixedSizeChoiceBuiltIn_BusCre/1  "<arr>"
  i36_SeqOfSeqOfSeqOfFixedSizeChoiceBuiltIn_BusSel/1 -> o36_SeqOfSeqOfSeqOfFixedSizeChoiceBuiltIn_BusCre/1  "<arr>"
  i20_SeqOfSeqOfFixedSizeOctetStringVarSizeAlias_BusSel1/1 -> o20_SeqOfSeqOfFixedSizeOctetStringVarSizeAlias_BusCre/1  "<arr>"
  i22_SeqOfFixedSizeEnumAlias_BusSel1/1 -> o22_SeqOfFixedSizeEnumAlias_BusCre/1  "<arr>"
  QgencimplseqoffixedsizeRi_Seqoffixedsizeiface/24 -> i24_SeqOfSeqOfSeqOfFixedSizeEnumAlias_BusSel1/1
  QgencimplseqoffixedsizeRi_Seqoffixedsizeiface/29 -> i29_SeqOfSeqOfFixedSizeSeqBuiltIn_BusSel1/1
  QgencimplseqoffixedsizeRi_Seqoffixedsizeiface/30 -> i30_SeqOfSeqOfSeqOfFixedSizeSeqBuiltIn_BusSel1/1
  QgencimplseqoffixedsizeRi_Seqoffixedsizeiface/9 -> i9_SeqOfSeqOfSeqOfFixedSizeRealAlias_BusSel1/1
  QgencimplseqoffixedsizeRi_Seqoffixedsizeiface/20 -> i20_SeqOfSeqOfFixedSizeOctetStringVarSizeAlias_BusSel1/1
  QgencimplseqoffixedsizeRi_Seqoffixedsizeiface/28 -> i28_SeqOfFixedSizeSeqBuiltIn_BusSel1/1
  QgencimplseqoffixedsizeRi_Seqoffixedsizeiface/26 -> i26_SeqOfSeqOfFixedSizeSeqAliases_BusSel1/1
  i25_SeqOfFixedSizeSeqAliases_BusSel1/1 -> o25_SeqOfFixedSizeSeqAliases_BusCre/1  "<arr>"
  QgencimplseqoffixedsizeRi_Seqoffixedsizeiface/25 -> i25_SeqOfFixedSizeSeqAliases_BusSel1/1
  QgencimplseqoffixedsizeRi_Seqoffixedsizeiface/8 -> i8_SeqOfSeqOfFixedSizeRealAlias_BusSel1/1
  QgencimplseqoffixedsizeRi_Seqoffixedsizeiface/18 -> i18_SeqOfSeqOfSeqOfFixedSizeOctetStringFixedSizeAlias_BusSel1/1
  QgencimplseqoffixedsizeRi_Seqoffixedsizeiface/10 -> i10_SeqOfFixedSizeIA5StringFixedSizeAlias_BusSel1/1
  QgencimplseqoffixedsizeRi_Seqoffixedsizeiface/22 -> i22_SeqOfFixedSizeEnumAlias_BusSel1/1
  QgencimplseqoffixedsizeRi_Seqoffixedsizeiface/13 -> i13_SeqOfFixedSizeIA5StringVarSizeAlias_BusSel1/1
  QgencimplseqoffixedsizeRi_Seqoffixedsizeiface/4 -> i4_SeqOfFixedSizeIntegerAlias_BusSel1/1
  QgencimplseqoffixedsizeRi_Seqoffixedsizeiface/2 -> i2_SeqOfSeqOfFixedSizeBoolAlias_BusSel1/1
  QgencimplseqoffixedsizeRi_Seqoffixedsizeiface/12 -> i12_SeqOfSeqOfSeqOfFixedSizeIA5StringFixedSizeAlias_BusSel1/1
  QgencimplseqoffixedsizeRi_Seqoffixedsizeiface/1 -> i1_SeqOfFixedSizeBoolAlias_BusSel1/1
  QgencimplseqoffixedsizeRi_Seqoffixedsizeiface/6 -> i6_SeqOfSeqOfSeqOfFixedSizeIntegerAlias_BusSel1/1
  QgencimplseqoffixedsizeRi_Seqoffixedsizeiface/27 -> i27_SeqOfSeqOfSeqOfFixedSizeSeqAliases_BusSel1/1
  i28_SeqOfFixedSizeSeqBuiltIn_BusSel1/1 -> o28_SeqOfFixedSizeSeqBuiltIn_BusCre/1  "<arr>"
  QgencimplseqoffixedsizeRi_Seqoffixedsizeiface/3 -> i3_SeqOfSeqOfSeqOfFixedSizeBoolAlias_BusSel1/1
  i30_SeqOfSeqOfSeqOfFixedSizeSeqBuiltIn_BusSel1/1 -> o30_SeqOfSeqOfSeqOfFixedSizeSeqBuiltIn_BusCre/1  "<arr>"
  QgencimplseqoffixedsizeRi_Seqoffixedsizeiface/19 -> i19_SeqOfFixedSizeOctetStringVarSizeAlias_BusSel1/1
  i29_SeqOfSeqOfFixedSizeSeqBuiltIn_BusSel1/1 -> o29_SeqOfSeqOfFixedSizeSeqBuiltIn_BusCre/1  "<arr>"
  QgencimplseqoffixedsizeRi_Seqoffixedsizeiface/7 -> i7_SeqOfFixedSizeRealAlias_BusSel1/1
  i12_SeqOfSeqOfSeqOfFixedSizeIA5StringFixedSizeAlias_BusSel1/1 -> o12_SeqOfSeqOfSeqOfFixedSizeIA5StringFixedSizeAlias_BusCre/1  "<arr>"
  i21_SeqOfSeqOfSeqOfFixedSizeOctetStringVarSizeAlias_BusSel1/1 -> o21_SeqOfSeqOfSeqOfFixedSizeOctetStringVarSizeAlias_BusCre/1  "<arr>"
  i11_SeqOfSeqOfFixedSizeIA5StringFixedSizeAlias_BusSel1/1 -> o11_SeqOfSeqOfFixedSizeIA5StringFixedSizeAlias_BusCre/1  "<arr>"
  QgencimplseqoffixedsizeRi_Seqoffixedsizeiface/17 -> i17_SeqOfSeqOfFixedSizeOctetStringFixedSizeAlias_BusSel1/1
  i10_SeqOfFixedSizeIA5StringFixedSizeAlias_BusSel1/1 -> o10_SeqOfFixedSizeIA5StringFixedSizeAlias_BusCre/1  "<arr>"
  QgencimplseqoffixedsizeRi_Seqoffixedsizeiface/16 -> i16_SeqOfFixedSizeOctetStringFixedSizeAlias_BusSel1/1
  i9_SeqOfSeqOfSeqOfFixedSizeRealAlias_BusSel1/1 -> o9_SeqOfSeqOfSeqOfFixedSizeRealAlias_BusCre/1  "<arr>"
  QgencimplseqoffixedsizeRi_Seqoffixedsizeiface/5 -> i5_SeqOfSeqOfFixedSizeIntegerAlias_BusSel1/1
  QgencimplseqoffixedsizeRi_Seqoffixedsizeiface/14 -> i14_SeqOfSeqOfFixedSizeIA5StringVarSizeAlias_BusSel1/1
  QgencimplseqoffixedsizeRi_Seqoffixedsizeiface/21 -> i21_SeqOfSeqOfSeqOfFixedSizeOctetStringVarSizeAlias_BusSel1/1
  i8_SeqOfSeqOfFixedSizeRealAlias_BusSel1/1 -> o8_SeqOfSeqOfFixedSizeRealAlias_BusCre/1  "<arr>"
  i5_SeqOfSeqOfFixedSizeIntegerAlias_BusSel1/1 -> o5_SeqOfSeqOfFixedSizeIntegerAlias_BusCre/1  "<arr>"
  i26_SeqOfSeqOfFixedSizeSeqAliases_BusSel1/1 -> o26_SeqOfSeqOfFixedSizeSeqAliases_BusCre/1  "<arr>"
  i16_SeqOfFixedSizeOctetStringFixedSizeAlias_BusSel1/1 -> o16_SeqOfFixedSizeOctetStringFixedSizeAlias_BusCre/1  "<arr>"
  i6_SeqOfSeqOfSeqOfFixedSizeIntegerAlias_BusSel1/1 -> o6_SeqOfSeqOfSeqOfFixedSizeIntegerAlias_BusCre/1  "<arr>"
  i2_SeqOfSeqOfFixedSizeBoolAlias_BusSel1/1 -> o2_SeqOfSeqOfFixedSizeBoolAlias_BusCre/1  "<arr>"
  QgencimplseqoffixedsizeRi_Seqoffixedsizeiface/23 -> i23_SeqOfSeqOfFixedSizeEnumAlias_BusSel1/1
  i4_SeqOfFixedSizeIntegerAlias_BusSel1/1 -> o4_SeqOfFixedSizeIntegerAlias_BusCre/1  "<arr>"
  i27_SeqOfSeqOfSeqOfFixedSizeSeqAliases_BusSel1/1 -> o27_SeqOfSeqOfSeqOfFixedSizeSeqAliases_BusCre/1  "<arr>"
  i1_SeqOfFixedSizeBoolAlias_BusSel1/1 -> o1_SeqOfFixedSizeBoolAlias_BusCre/1  "<arr>"
  i17_SeqOfSeqOfFixedSizeOctetStringFixedSizeAlias_BusSel1/1 -> o17_SeqOfSeqOfFixedSizeOctetStringFixedSizeAlias_BusCre/1  "<arr>"
  i18_SeqOfSeqOfSeqOfFixedSizeOctetStringFixedSizeAlias_BusSel1/1 -> o18_SeqOfSeqOfSeqOfFixedSizeOctetStringFixedSizeAlias_BusCre/1  "<arr>"
  i14_SeqOfSeqOfFixedSizeIA5StringVarSizeAlias_BusSel1/1 -> o14_SeqOfSeqOfFixedSizeIA5StringVarSizeAlias_BusCre/1  "<arr>"
  i13_SeqOfFixedSizeIA5StringVarSizeAlias_BusSel1/1 -> o13_SeqOfFixedSizeIA5StringVarSizeAlias_BusCre/1  "<arr>"
  QgencimplseqoffixedsizeRi_Seqoffixedsizeiface/11 -> i11_SeqOfSeqOfFixedSizeIA5StringFixedSizeAlias_BusSel1/1
  i3_SeqOfSeqOfSeqOfFixedSizeBoolAlias_BusSel1/1 -> o3_SeqOfSeqOfSeqOfFixedSizeBoolAlias_BusCre/1  "<arr>"
  i7_SeqOfFixedSizeRealAlias_BusSel1/1 -> o7_SeqOfFixedSizeRealAlias_BusCre/1  "<arr>"
  QgencimplseqoffixedsizeRi_Seqoffixedsizeiface/15 -> i15_SeqOfSeqOfSeqOfFixedSizeIA5StringVarSizeAlias_BusSel1/1
  i23_SeqOfSeqOfFixedSizeEnumAlias_BusSel1/1 -> o23_SeqOfSeqOfFixedSizeEnumAlias_BusCre/1  "<arr>"
  i24_SeqOfSeqOfSeqOfFixedSizeEnumAlias_BusSel1/1 -> o24_SeqOfSeqOfSeqOfFixedSizeEnumAlias_BusCre/1  "<arr>"
  i19_SeqOfFixedSizeOctetStringVarSizeAlias_BusSel1/1 -> o19_SeqOfFixedSizeOctetStringVarSizeAlias_BusCre/1  "<arr>"
  i15_SeqOfSeqOfSeqOfFixedSizeIA5StringVarSizeAlias_BusSel1/1 -> o15_SeqOfSeqOfSeqOfFixedSizeIA5StringVarSizeAlias_BusCre/1  "<arr>"
